simulink model "TCMSSystem"  (R2019b)
settings: configuration reference "ConfigSet_TCMSSystem_Reference" (kept outside this file)
model workspace (MAT data in the model file):
  Prm_TCMSSystem : Simulink.Parameter (value not decoded)
  SampleTime = 0.05
symbols that are objects in the model workspace (value not decoded): Prm_TCMSSystem
undefined symbols (not defined in the file): ADDIntervention, AK1Status, AK2Status, AKContactorStatus, AllDoorsClosed, AllLeftDoorsClosed, AllRightDoorsClosed, APS1Fault, APS1Isolated, APS1OutputVoltage, APS1Status, APS2Fault, APS2Isolated, APS2OutputVoltage, APS2Status, APSKAKContactor, ASCOEnd1, ASCOEnd2, ATBMode, ATCBypassMode, ATCStatusNotOK, ATOMode, ATPLowSpeedCutoutStatus, ATPMode, AuxCompressor, BatteryCurrent, BatteryIsolationContactor, BatteryTemperature, BatteryVoltage, BCG1Fault, BCG1Isolated, BCG1IsolationFailed, BCG1OutputCurrent, BCG1Status, BCG2Fault, BCG2Isolated, BCG2OutputCurrent, BCG2Status, BCGOutputVoltage, BECU1AxleLockedWheelSet1, BECU2AxleLockedWheelSet2, BECUFaulty, BECUMajorFault, BECUMinorFault, BECUStatus, BIC1Inside, BIC1Outside, BIC2Inside, BIC2Outside, Bogie, Bogie1WSPStatus, Bogie2WSPStatus, BogieFaulty, BogieIsolationStatus, BogieSupportedMass, BrakeCylinderPressureGauge, BrakeLoopCBTripped, BrakeLoopOpenTL, BrakeTrainLineStatus, BrakingDemand ... (+215)
libraries: TimersLib x257, simulink x137, LatchesLib x42, VectorOperationsLib x15, TestBenchLib x12, MathOperationsLib x2, FiltersLib x1
(part 7 of 16)

== system TCMSSystem/TCMSSystemPerVehicle/EnabledTCMSVehicle/TCMSTractionBraking/TractionBrakingControl/ForEachBogie ==
  BECUFault : Inport
  BogieBrakingEffortDemand : Inport  Port=2
  DisplayBogieControl : Inport  Port=3  Partition=on  PartitionDimension=1  PartitionWidth=1  PartitionOffset=0
  TractionBrakingBogieData : Inport  Port=4  Partition=on  PartitionDimension=1  PartitionWidth=1  PartitionOffset=0
  BogieIsolationStatus : Inport  Port=5  Partition=on  PartitionDimension=1  PartitionWidth=1  PartitionOffset=0
  UnitData : Inport  Port=6
  DynamicsIn : Inport  Port=7
  Bus Assignment : BusAssignment  AssignedSignals=EPBrakingDemand,TractionInhibit,EDBrakingInhibit,BogieSupportedMass,BogieIsolationStatus
  Bus Selector : BusSelector  OutputSignals=EstimatedSupportedMass
  Bus Selector1 : BusSelector  OutputSignals=TractionInhibit,EDBrakingInhibit
  Bus Selector2 : BusSelector  OutputSignals=EDBrakingEffortAchieved
  Constant : Constant  Value=0
  Constant7 : Constant  Value=0  OutDataTypeStr=Bus: BD_TCMSSystem_Out_Vehicle_Control_TractionBraking_Bogie
  For Each : ForEach  DisableCoverage=on
  Subsystem : Subsystem
  Sum : Sum  Inputs=+-
  Switch : Switch  Criteria=u2 > Threshold
  Terminator : Terminator
  BogieControl : Outport  ConcatenationDimension=1
  wires:
  TractionBrakingBogieData/1 -> Subsystem/3(EffortsAchivedPerVehicle), Bus Selector2/1, Bus Selector/1
  DisplayBogieControl/1 -> Bus Selector1/1
  Constant7/1 -> Bus Assignment/1  "Control"
  Bus Selector1/1 -> Bus Assignment/3  "<TractionInhibit>"
  Bus Selector1/2 -> Bus Assignment/4  "<EDBrakingInhibit>"
  Bus Selector/1 -> Bus Assignment/5  "<EstimatedSupportedMass>"
  Bus Assignment/1 -> BogieControl/1  "Control"
  BECUFault/1 -> Switch/2
  Constant/1 -> Switch/1
  Switch/1 -> Bus Assignment/2
  BogieIsolationStatus/1 -> Bus Assignment/6
  UnitData/1 -> Subsystem/1(EffortsAchievedPerUnit)
  DynamicsIn/1 -> Subsystem/2(Speed)
  BogieBrakingEffortDemand/1 -> Sum/1
  Bus Selector2/1 -> Sum/2  "<EDBrakingEffortAchieved>"
  Sum/1 -> Switch/3
  Subsystem/1(SelectEPBrakeDemand) -> Terminator/1

== system TCMSSystem/TCMSSystemPerVehicle/EnabledTCMSVehicle/TCMSTractionBraking/TractionBrakingControl/NonCabTWsAssignment ==
  TractionForce : Inport
  TractionBrakingTrainWireSource : Inport  Port=2
  EstimatedMass : Inport  Port=3
  Bus Assignment1 : BusAssignment  AssignedSignals=EstimatedMass,TractionForce
  Control : Outport
  wires:
  TractionBrakingTrainWireSource/1 -> Bus Assignment1/1
  EstimatedMass/1 -> Bus Assignment1/2
  Bus Assignment1/1 -> Control/1  "Control"
  TractionForce/1 -> Bus Assignment1/3

== system TCMSSystem/TCMSSystemPerVehicle/EnabledTCMSVehicle/TCMSTractionBraking/TractionBrakingControl/Subsystem ==
  <EstimatedSupportedMass> : Inport  Partition=on  PartitionDimension=1  PartitionWidth=1  PartitionOffset=0
  Bus Selector1 : BusSelector  OutputSignals=EstimatedSupportedMass
  For Each : ForEach  DisableCoverage=on
  EstimatedMassPerVehicle : Outport  ConcatenationDimension=1
  wires:
  <EstimatedSupportedMass>/1 -> Bus Selector1/1
  Bus Selector1/1 -> EstimatedMassPerVehicle/1  "<EstimatedSupportedMass>"

== system TCMSSystem/TCMSSystemPerVehicle/EnabledTCMSVehicle/TCMSTractionBraking/TractionBrakingControl/Subsystem1 ==
  In1 : Inport  Partition=on  PartitionDimension=1  PartitionWidth=1  PartitionOffset=0
  Bus Selector7 : BusSelector  OutputSignals=SpeedSensorFault
  For Each : ForEach  DisableCoverage=on
  <SpeedSensorFault> : Outport  ConcatenationDimension=1
  wires:
  In1/1 -> Bus Selector7/1
  Bus Selector7/1 -> <SpeedSensorFault>/1  "<SpeedSensorFault>"

== system TCMSSystem/TCMSSystemPerVehicle/EnabledTCMSVehicle/TCMSTractionBraking/TractionBrakingControl/Subsystem15 ==
  Fault : Inport
  ClearCond : Inport  Port=2
  Data Type Conversion : DataTypeConversion
  SR Latch - Reset Priority : LatchesLib/SR Latch - Reset Priority  initial_condition=0
      settings: SourceProductName=Latches
  Trig : Outport
  wires:
  Fault/1 -> SR Latch - Reset Priority/1
  SR Latch - Reset Priority/1 -> Data Type Conversion/1
  ClearCond/1 -> SR Latch - Reset Priority/2
  Data Type Conversion/1 -> Trig/1

== system TCMSSystem/TCMSSystemPerVehicle/EnabledTCMSVehicle/TCMSTractionBraking/TractionBrakingControl/Subsystem2 ==
  Fault : Inport
  ClearCond : Inport  Port=2
  Data Type Conversion : DataTypeConversion
  SR Latch - Reset Priority : LatchesLib/SR Latch - Reset Priority  initial_condition=0
      settings: SourceProductName=Latches
  Trig : Outport
  wires:
  Data Type Conversion/1 -> Trig/1
  ClearCond/1 -> SR Latch - Reset Priority/2
  SR Latch - Reset Priority/1 -> Data Type Conversion/1
  Fault/1 -> SR Latch - Reset Priority/1

== system TCMSSystem/TCMSSystemPerVehicle/EnabledTCMSVehicle/TCMSTractionBraking/TractionBrakingControl/Subsystem3 ==
  In1 : Inport  Partition=on  PartitionDimension=1  PartitionWidth=1  PartitionOffset=0
  Bus Selector7 : BusSelector  OutputSignals=TCUSlideDetected,TCUSlipDetected
  For Each : ForEach  DisableCoverage=on
  Logical Operator : Logic  Operator=OR  AllPortsSameDT=off  OutDataTypeStr=boolean
  SlipSlideDetected : Outport  ConcatenationDimension=1
  wires:
  Bus Selector7/1 -> Logical Operator/1  "<TCUSlideDetected>"
  In1/1 -> Bus Selector7/1
  Logical Operator/1 -> SlipSlideDetected/1
  Bus Selector7/2 -> Logical Operator/2  "<TCUSlipDetected>"

== system TCMSSystem/TCMSSystemPerVehicle/EnabledTCMSVehicle/TCMSTractionBraking/TractionBrakingControl/Subsystem4 ==
  In1 : Inport
  Bus Selector9 : BusSelector  OutputSignals=Bogie1IsolationCmd,Bogie2IsolationCmd
  Mux : Mux  Inputs=2
  Out1 : Outport
  wires:
  Bus Selector9/1 -> Mux/1  "<Bogie1IsolationCmd>"
  Bus Selector9/2 -> Mux/2  "<Bogie2IsolationCmd>"
  In1/1 -> Bus Selector9/1
  Mux/1 -> Out1/1

== system TCMSSystem/TCMSSystemPerVehicle/EnabledTCMSVehicle/TCMSTractionBraking/TractionBrakingDataExtract/Subsystem ==
  BogieData : Inport  Partition=on  PartitionDimension=1  PartitionWidth=1  PartitionOffset=0
  Bus Selector1 : BusSelector  OutputSignals=TCUStatus
  For Each : ForEach  DisableCoverage=on
  <TCUStatus> : Outport  ConcatenationDimension=1
  wires:
  Bus Selector1/1 -> <TCUStatus>/1  "<TCUStatus>"
  BogieData/1 -> Bus Selector1/1

== system TCMSSystem/TCMSSystemPerVehicle/EnabledTCMSVehicle/TCMSTractionBraking/TractionBrakingDataExtract/TCMSTractionBogie ==
  TractionBogieSignals : Inport  Partition=on  PartitionDimension=1  PartitionWidth=1  PartitionOffset=0
  PneumaticsBogieSignals : Inport  Port=2  Partition=on  PartitionDimension=1  PartitionWidth=1  PartitionOffset=0
  Bus Assignment : BusAssignment  AssignedSignals=TCUStatus,BogieFaulty,TractionNotIsolated,EDBrakeNotIsolated,TCUSlideDetected,TCUSlipDetected,TractiveEffortAchieved,EDBrakingEffortAchieved,TractiveEffortPossible,EDBrakingEffortPossible,TractionPower,EDBrakingPower,TractivePowerPossible,EDBrakingPowerPossible,MotorSpeeds,ASPressureSwitchStatus,EstimatedSupportedMass
  Bus Selector : BusSelector  OutputSignals=TCUStatus,BogieFaulty,TractionNotIsolated,EDBrakeNotIsolated,TCUSlideDetected,TCUSlipDetected,TractiveEffortAchieved,EDBrakingEffortAchieved,TractiveEffortPossible,EDBrakingEffortPossible,TractionPower,EDBrakingPower,TractivePowerPossible,EDBrakingPowerPossible,MotorSpeeds
  Bus Selector1 : BusSelector  OutputSignals=AirSuspensionSwitchStatus,AirSuspensionLoadPressure
  Constant : Constant  Value=Prm_TCMSSystem.LoadCompensationMasses
  Constant1 : Constant  Value=Prm_TCMSSystem.LoadCompensationPressures
  Constant7 : Constant  Value=0  OutDataTypeStr=Bus: BD_TCMSSystem_Out_Vehicle_Display_TractionBraking_Bogie
  Data Type Conversion{,1..14} (15 alike) : DataTypeConversion  OutDataTypeStr=double
  For Each : ForEach  DisableCoverage=on
  Lookup Table Dynamic : simulink/Lookup Tables/Lookup Table Dynamic  LookUpMeth=Interpolation-Use End Values  OutDataType=fixdt('double')  OutScaling=[]  OutputDataTypeScalingMode=Specify via dialog  OutDataTypeStr=double  DoSatur=off
      settings: SourceProductName=Simulink
  TCMSBogieData : Outport  ConcatenationDimension=1
  BogieTractiveEffortAchieved : Outport  Port=2  ConcatenationDimension=1
  BogieEDBrakingEffortAchieved : Outport  Port=3  ConcatenationDimension=1
  BogieTractiveEffortPossible : Outport  Port=4  ConcatenationDimension=1
  BogieEDBrakingEffortPossible : Outport  Port=5  ConcatenationDimension=1
  BogieTractivePowerAchieved : Outport  Port=6  ConcatenationDimension=1
  BogieEDBrakingPowerAchieved : Outport  Port=7  ConcatenationDimension=1
  BogieTractivePowerPossible : Outport  Port=8  ConcatenationDimension=1
  BogieEDBrakingPowerPossible : Outport  Port=9  ConcatenationDimension=1
  EstimatedBogieSupportedMass : Outport  Port=10  ConcatenationDimension=1
  TractionBogieAvailable : Outport  Port=11  ConcatenationDimension=1
  EDBrakingBogieAvailable : Outport  Port=12  ConcatenationDimension=1
  BogieFaulty : Outport  Port=13  ConcatenationDimension=1
  wires:
  Data Type Conversion3/1 -> Bus Assignment/6
  Bus Selector/15 -> Data Type Conversion8/1  "<MotorSpeeds>"
  Bus Selector/5 -> Data Type Conversion3/1  "<TCUSlideDetected>"
  Data Type Conversion10/1 -> BogieTractivePowerPossible/1, Bus Assignment/14
  Bus Selector/1 -> Data Type Conversion7/1  "<TCUStatus>"
  TractionBogieSignals/1 -> Bus Selector/1
  Bus Selector/10 -> Data Type Conversion13/1  "<EDBrakingEffortPossible>"
  Data Type Conversion13/1 -> Bus Assignment/11, BogieEDBrakingEffortPossible/1
  Bus Selector/13 -> Data Type Conversion10/1  "<TractivePowerPossible>"
  Bus Selector/12 -> Data Type Conversion11/1  "<EDBrakingPower>"
  Bus Selector/14 -> Data Type Conversion9/1  "<EDBrakingPowerPossible>"
  Bus Selector/6 -> Data Type Conversion2/1  "<TCUSlipDetected>"
  Data Type Conversion5/1 -> Bus Assignment/4, TractionBogieAvailable/1
  Bus Selector/11 -> Data Type Conversion12/1  "<TractionPower>"
  Bus Selector/4 -> Data Type Conversion4/1  "<EDBrakeNotIsolated>"
  Data Type Conversion9/1 -> BogieEDBrakingPowerPossible/1, Bus Assignment/15
  Data Type Conversion12/1 -> BogieTractivePowerAchieved/1, Bus Assignment/12
  Data Type Conversion2/1 -> Bus Assignment/7
  Bus Selector/9 -> Data Type Conversion14/1  "<TractiveEffortPossible>"
  Data Type Conversion14/1 -> Bus Assignment/10, BogieTractiveEffortPossible/1
  Data Type Conversion/1 -> Bus Assignment/9, BogieEDBrakingEffortAchieved/1
  Constant7/1 -> Bus Assignment/1  "Display"
  Bus Selector/8 -> Data Type Conversion/1  "<EDBrakingEffortAchieved>"
  Data Type Conversion8/1 -> Bus Assignment/16
  Bus Selector/3 -> Data Type Conversion5/1  "<TractionNotIsolated>"
  Bus Selector/2 -> Data Type Conversion6/1  "<BogieFaulty>"
  Data Type Conversion7/1 -> Bus Assignment/2
  Data Type Conversion6/1 -> BogieFaulty/1, Bus Assignment/3
  Bus Selector/7 -> Data Type Conversion1/1  "<TractiveEffortAchieved>"
  Bus Assignment/1 -> TCMSBogieData/1  "Display"
  Data Type Conversion1/1 -> Bus Assignment/8, BogieTractiveEffortAchieved/1
  Data Type Conversion4/1 -> EDBrakingBogieAvailable/1, Bus Assignment/5
  Data Type Conversion11/1 -> Bus Assignment/13, BogieEDBrakingPowerAchieved/1
  PneumaticsBogieSignals/1 -> Bus Selector1/1
  Bus Selector1/2 -> Lookup Table Dynamic/1  "<AirSuspensionLoadPressure>"
  Constant1/1 -> Lookup Table Dynamic/2
  Constant/1 -> Lookup Table Dynamic/3
  Lookup Table Dynamic/1 -> Bus Assignment/18, EstimatedBogieSupportedMass/1
  Bus Selector1/1 -> Bus Assignment/17  "<AirSuspensionSwitchStatus>"

== system TCMSSystem/TCMSSystemPerVehicle/EnabledTCMSVehicle/TCMSTractionBraking/TractionBrakingDisplay/BrakeScreen ==
  note: Instead of making the fault on bogie level, we only change
      | the icon at bogie level to make it simpler.
  note: Added as per BEML requirements
  note: BrakeScreen
  note: Isolation status 0 means not isolated.
  note: BECU Status is currently mapped to
      | TCUStatus(via PropulsionEnabled)
      | which is actually TCU Power
  BusIn : Inport
  In Bus Element14 : Inport  Port=2  PortName=TractionBrakingTW  Element=HoldingBrakeStatus
  In Bus Element16 : Inport  Port=2  PortName=TractionBrakingTW  Element=EstimatedMass
  In Bus Element9 : Inport  Port=3  PortName=IOControl  Element=EPIC
  In Bus Element12 : Inport  Port=3  PortName=IOControl  Element=SR
  In Bus Element13 : Inport  Port=4  PortName=TractionVehicleData  Element=EstimatedMass
  In Bus Element1 : Inport  Port=5  PortName=TractionOnBogieData
  In Bus Element17 : Inport  Port=6  PortName=BrakingSystem  Element=BrakingForce
  In Bus Element2 : Inport  Port=7  PortName=ElectricalSignals  Element=BCUPower
  In Bus Element3 : Inport  Port=8  PortName=Faults  Element=DynamicBrakeCutOut
  In Bus Element4 : Inport  Port=8  PortName=Faults  Element=BECUMajorFault
  In Bus Element5 : Inport  Port=8  PortName=Faults  Element=BECUMajorFaultWired
  In Bus Element7 : Inport  Port=9  PortName=VehicleFaults  Element=BECU1ServiceBrakeFailure
  In Bus Element8 : Inport  Port=9  PortName=VehicleFaults  Element=BECU1EmergencyBrakeFailure
  In Bus Element10 : Inport  Port=9  PortName=VehicleFaults  Element=BECU2EmergencyBrakeFailure
  In Bus Element6 : Inport  Port=9  PortName=VehicleFaults  Element=WSPActiveBogie1
  In Bus Element : Inport  Port=9  PortName=VehicleFaults  Element=BECU2MinorFault
  In Bus Element15 : Inport  Port=9  PortName=VehicleFaults  Element=BECULowRPressure
  In Bus Element18 : Inport  Port=9  PortName=VehicleFaults  Element=BECU2CarLoadPressureLow
  In Bus Element11 : Inport  Port=9  PortName=VehicleFaults  Element=BECU1CarLoadPressureLow
  AND : Logic  AllPortsSameDT=off  OutDataTypeStr=boolean
  Bus Assignment9 : BusAssignment  AssignedSignals=HoldingBrakeStatus,EPICIsolationStatus,RPRESSIsolationStatus,CarWeight,TotalWeight,Bogie1WSPStatus,Bogie2WSPStatus,EPBrakeDelivered,EDBrakeRequested,BECUStatus,BECUMinorFault,BECUMajorFault,EDCutoutStatus,DynamicBrakeCutoutDueToSlide
  Data Type Conversion{1..10} (10 alike) : DataTypeConversion
  Demux : Demux  Outputs=2
  For Each Subsystem : Subsystem  TreatAsAtomicUnit=on
  Logical Operator : Logic  Operator=OR  Inputs=4  AllPortsSameDT=off  OutDataTypeStr=boolean
  Logical Operator1 : Logic  Operator=NOT  AllPortsSameDT=off  OutDataTypeStr=boolean
  Logical Operator2 : Logic  Operator=NOT  AllPortsSameDT=off  OutDataTypeStr=boolean
  Logical Operator3 : Logic  Operator=NOT  AllPortsSameDT=off  OutDataTypeStr=boolean
  Logical Operator5 : Logic  Operator=OR  Inputs=1  AllPortsSameDT=off  OutDataTypeStr=boolean
  NOT : Logic  Operator=NOT  AllPortsSameDT=off  OutDataTypeStr=boolean
  OR : Logic  Inputs=1  AllPortsSameDT=off  OutDataTypeStr=boolean
  OR1 : Logic  Operator=OR  Inputs=5  AllPortsSameDT=off  OutDataTypeStr=boolean
  OR2 : Logic  AllPortsSameDT=off  OutDataTypeStr=boolean
  BusOut : Outport
  tag scope: SlipDetected=scoped
  wires:
  Bus Assignment9/1 -> BusOut/1
  BusIn/1 -> Bus Assignment9/1
  In Bus Element14/1 -> Data Type Conversion2/1
  Data Type Conversion2/1 -> Bus Assignment9/2
  Data Type Conversion1/1 -> Bus Assignment9/4
  In Bus Element12/1 -> Logical Operator2/1
  Logical Operator1/1 -> Data Type Conversion5/1
  Data Type Conversion5/1 -> Bus Assignment9/3
  In Bus Element9/1 -> Logical Operator1/1
  Logical Operator2/1 -> Data Type Conversion1/1
  In Bus Element13/1 -> Bus Assignment9/5
  In Bus Element16/1 -> Bus Assignment9/6
  For Each Subsystem/2(SlipDetected) -> Logical Operator5/1
  Logical Operator5/1 -> [SlipDetected]
  In Bus Element1/1 -> For Each Subsystem/1(In1)
  Demux/1 -> Bus Assignment9/7
  For Each Subsystem/1(SlideDetected) -> Data Type Conversion4/1
  Demux/2 -> OR2/1
  In Bus Element17/1 -> Bus Assignment9/9
  [EDBrakeRequested] -> Bus Assignment9/10
  Data Type Conversion10/1 -> Bus Assignment9/12
  Data Type Conversion6/1 -> Bus Assignment9/11
  In Bus Element2/1 -> Data Type Conversion6/1
  For Each Subsystem/3(EDBrakeAvailable) -> OR/1
  OR/1 -> NOT/1
  Data Type Conversion3/1 -> Bus Assignment9/14
  NOT/1 -> Data Type Conversion3/1, AND/1
  Data Type Conversion4/1 -> Demux/1
  In Bus Element3/1 -> AND/2
  AND/1 -> Data Type Conversion7/1
  Data Type Conversion7/1 -> Bus Assignment9/15
  OR1/1 -> Data Type Conversion8/1
  In Bus Element4/1 -> OR1/1
  In Bus Element5/1 -> OR1/2
  Data Type Conversion8/1 -> Bus Assignment9/13
  In Bus Element7/1 -> OR1/3
  In Bus Element8/1 -> OR1/4
  In Bus Element10/1 -> OR1/5
  In Bus Element6/1 -> Logical Operator3/1
  Logical Operator3/1 -> OR2/2
  OR2/1 -> Data Type Conversion9/1
  Data Type Conversion9/1 -> Bus Assignment9/8
  In Bus Element18/1 -> Logical Operator/3
  In Bus Element15/1 -> Logical Operator/2
  In Bus Element/1 -> Logical Operator/1
  Logical Operator/1 -> Data Type Conversion10/1
  In Bus Element11/1 -> Logical Operator/4

== system TCMSSystem/TCMSSystemPerVehicle/EnabledTCMSVehicle/TCMSTractionBraking/TractionBrakingDisplay/HVScreen ==
  note: HighVoltageScreen
  In Bus Element5 : Inport  PortName=BusIn
  In Bus Element1 : Inport  Port=2  PortName=ElectricalSignals  Element=UW_VCB
  In Bus Element : Inport  Port=2  PortName=ElectricalSignals  Element=VCBI_KAKContactorCI
  In Bus Element27 : Inport  Port=3  PortName=TractionBrakingUW  Element=CI_K_AK_Status
  Bus Assignment9 : BusAssignment  AssignedSignals=CIStatus,CIKAKContactor
  Data Type Conversion7 : DataTypeConversion
  Logical Operator : Logic  Operator=OR  AllPortsSameDT=off  OutDataTypeStr=boolean
  Display : Outport
  wires:
  In Bus Element5/1 -> Bus Assignment9/1
  Bus Assignment9/1 -> Display/1  "Display"
  In Bus Element1/1 -> Bus Assignment9/2
  Data Type Conversion7/1 -> Bus Assignment9/3
  Logical Operator/1 -> Data Type Conversion7/1
  In Bus Element27/1 -> Logical Operator/1
  In Bus Element/1 -> Logical Operator/2

== system TCMSSystem/TCMSSystemPerVehicle/EnabledTCMSVehicle/TCMSTractionBraking/TractionBrakingDisplay/OperatingandOtherScreen ==
  note: OperatingandOtherScreen
  BusIn : Inport
  In Bus Element2 : Inport  Port=2  PortName=TCMSSystemVehicleConfig
  In Bus Element : Inport  Port=3  PortName=ElectricalSignals
  In Bus Element21 : Inport  Port=4  PortName=TractionUnitData
  In Bus Element5 : Inport  Port=5  PortName=TractionVehicleData
  In Bus Element15 : Inport  Port=6  PortName=TractionBrakingTW  Element=TCMSSpeedLimit
  Abs : Abs
  Bus Assignment : BusAssignment  AssignedSignals=ForwardDirection,ReverseDirection,TrainSpeed,ZeroSpeed,TractionOn,BrakeOn,TractionSafe,UnitTractiveEffortAchieved,UnitTractiveEffortPossible,UnitEDBrakingEffortAchieved,UnitEDBrakingEffortPossible,UnitTractivePower,UnitTractivePowerPossible,UnitEDBrakingPower,UnitEDBrakingPowerPossible,VehicleTractiveEffortPossible,VehicleEDBrakingEffortAchieved,VehicleEDBrakingEffortPossible,VehicleTractivePower,VehicleTractivePowerPossible,VehicleEDBrakingPower,VehicleEDBrakingPowerPossible,VehicleTractiveEffortAchieved,TractiveEffort,TCMSSpeedLimit
  Bus Selector : BusSelector  OutputSignals=TractiveEffortPossible,EDBrakingEffortAchieved,EDBrakingEffortPossible,TractivePowerAchieved,TractivePowerPossible,EDBrakingPowerAchieved,EDBrakingPowerPossible,TractiveEffortAchieved
  Bus Selector1 : BusSelector  OutputSignals=ForwardDirection,ReverseDirection,Speedometer,ZeroSpeed,TractionOn,BrakeOn,TractionSafe,UnitTractiveEffortAchieved,UnitEDBrakingEffortAchieved,UnitTractiveEffortPossible,UnitEDBrakingEffortPossible,UnitTractivePowerAchieved,UnitEDBrakingPowerAchieved,UnitTractivePowerPossible,UnitEDBrakingPowerPossible
  CabUnitDisplay : Subsystem
  BusOut : Outport
  wires:
  Bus Selector1/6 -> Bus Assignment/7  "<BrakeOn>"
  BusIn/1 -> Bus Assignment/1  "Display"
  Bus Selector1/10 -> Bus Assignment/11  "<UnitTractiveEffortPossible>"
  Bus Selector1/3 -> Bus Assignment/4  "<Speedometer>"
  Bus Selector/6 -> Bus Assignment/22  "<EDBrakingPowerAchieved>"
  Bus Selector1/12 -> Bus Assignment/13  "<UnitTractivePowerAchieved>"
  Bus Assignment/1 -> BusOut/1
  Bus Selector/1 -> Bus Assignment/17  "<TractiveEffortPossible>"
  Bus Selector1/15 -> Bus Assignment/16  "<UnitEDBrakingPowerPossible>"
  Bus Selector1/7 -> Bus Assignment/8  "<TractionSafe>"
  Bus Selector1/2 -> Bus Assignment/3  "<ReverseDirection>"
  Bus Selector1/5 -> Bus Assignment/6  "<TractionOn>"
  Bus Selector1/14 -> Bus Assignment/15  "<UnitTractivePowerPossible>"
  Bus Selector1/8 -> Bus Assignment/9  "<UnitTractiveEffortAchieved>"
  Bus Selector1/1 -> Bus Assignment/2  "<ForwardDirection>"
  Bus Selector/4 -> Bus Assignment/20  "<TractivePowerAchieved>"
  Bus Selector1/11 -> Bus Assignment/12  "<UnitEDBrakingEffortPossible>"
  Bus Selector/2 -> Bus Assignment/18  "<EDBrakingEffortAchieved>"
  Bus Selector/3 -> Bus Assignment/19  "<EDBrakingEffortPossible>"
  CabUnitDisplay/1(CabUnitDisplay) -> Bus Selector1/1
  Bus Selector/7 -> Bus Assignment/23  "<EDBrakingPowerPossible>"
  Bus Selector1/13 -> Bus Assignment/14  "<UnitEDBrakingPowerAchieved>"
  Bus Selector1/9 -> Bus Assignment/10  "<UnitEDBrakingEffortAchieved>"
  Bus Selector1/4 -> Bus Assignment/5  "<ZeroSpeed>"
  Bus Selector/8 -> Abs/1  "<TractiveEffortAchieved>"
  Bus Selector/5 -> Bus Assignment/21  "<TractivePowerPossible>"
  In Bus Element2/1 -> CabUnitDisplay/1(TCMSConfig)
  In Bus Element/1 -> CabUnitDisplay/2(ElectricalSignals)
  In Bus Element21/1 -> CabUnitDisplay/3(TractionUnitData)
  In Bus Element5/1 -> Bus Selector/1
  Abs/1 -> Bus Assignment/25, Bus Assignment/24
  In Bus Element15/1 -> Bus Assignment/26

== system TCMSSystem/TCMSSystemPerVehicle/EnabledTCMSVehicle/TCMSTractionBraking/TractionBrakingDisplay/PropulsionScreen ==
  note: PropulsionScreen
  BusIn : Inport
  In Bus Element24 : Inport  Port=2  PortName=TractionBrakingUnitData  Element=PropulsionFault
  In Bus Element26 : Inport  Port=2  PortName=TractionBrakingUnitData  Element=PropulsionEnabled
  In Bus Element8 : Inport  Port=2  PortName=TractionBrakingUnitData  Element=PropulsionActive
  In Bus Element18 : Inport  Port=3  PortName=TractionSystem  Element=TCU_KStatus
  In Bus Element19 : Inport  Port=3  PortName=TractionSystem  Element=TCU_AKStatus
  In Bus Element20 : Inport  Port=3  PortName=TractionSystem  Element=FilterVoltage
  In Bus Element1 : Inport  Port=3  PortName=TractionSystem  Element=Bogie
  In Bus Element : Inport  Port=4  PortName=TractionOnBogieData
  In Bus Element4 : Inport  Port=5  PortName=ElectricalFB  Element=CIIsolated
  In Bus Element9 : Inport  Port=5  PortName=ElectricalFB  Element=CIIsolated
  In Bus Element5 : Inport  Port=5  PortName=ElectricalFB  Element=CabActive
  In Bus Element3 : Inport  Port=6  PortName=VehicleFault  Element=CIFailure
  In Bus Element10 : Inport  Port=6  PortName=VehicleFault  Element=LineConverterIGBTFailure
  In Bus Element2 : Inport  Port=7  PortName=CBTC  Element=RollbackDetected
  In Bus Element6 : Inport  Port=8  PortName=TractionTW  Element=HTERequired
  In Bus Element7 : Inport  Port=8  PortName=TractionTW  Element=WashModeActive
  In Bus Element11 : Inport  Port=8  PortName=TractionTW  Element=ShuntModeActive
  In Bus Element12 : Inport  Port=8  PortName=TractionTW  Element=ATPLowSpeedCutoutModeActive
  Bus Assignment9 : BusAssignment  AssignedSignals=PropulsionActive,PropulsionFault,CIFault,PropulsionIsolated,PropulsionEnableStatus,KContactorStatus,AKContactorStatus,FilterVoltage,EDBrakeStatus,HeavyWheelSlipDetected,RollbackDetected,HTERequired,WashingModeStatus,CIIsolated,ShuntModeStatus,ATPLowSpeedCutoutStatus
  Data Type Conversion{1..6} (6 alike) : DataTypeConversion
  For Each Subsystem : Subsystem  TreatAsAtomicUnit=on
  Logical Operator : Logic  Operator=OR  Inputs=3  AllPortsSameDT=off  OutDataTypeStr=boolean
  Logical Operator1 : Logic  AllPortsSameDT=off  OutDataTypeStr=boolean
  Logical Operator2 : Logic  Operator=NOT  AllPortsSameDT=off  OutDataTypeStr=boolean
  Logical Operator3 : Logic  AllPortsSameDT=off  OutDataTypeStr=boolean
  OR : Logic  Inputs=1  AllPortsSameDT=off  OutDataTypeStr=boolean
  OR1 : Logic  Operator=OR  Inputs=1  AllPortsSameDT=off  OutDataTypeStr=boolean
  BusOut : Outport
  wires:
  BusIn/1 -> Bus Assignment9/1
  Bus Assignment9/1 -> BusOut/1
  In Bus Element24/1 -> Logical Operator/1
  In Bus Element4/1 -> Logical Operator2/1, Bus Assignment9/5
  In Bus Element26/1 -> Bus Assignment9/6
  In Bus Element8/1 -> Bus Assignment9/2
  In Bus Element20/1 -> Bus Assignment9/9
  Data Type Conversion2/1 -> Bus Assignment9/7
  Data Type Conversion3/1 -> Bus Assignment9/8
  In Bus Element19/1 -> Data Type Conversion3/1
  In Bus Element18/1 -> Data Type Conversion2/1
  Data Type Conversion4/1 -> Bus Assignment9/10
  OR/1 -> Data Type Conversion4/1
  For Each Subsystem/1(EDBrakeAvailable) -> OR/1
  In Bus Element/1 -> For Each Subsystem/1(In1)
  In Bus Element1/1 -> For Each Subsystem/2(In2)
  For Each Subsystem/2(HeavyWheelSlipDetected) -> OR1/1
  OR1/1 -> Data Type Conversion1/1
  Data Type Conversion1/1 -> Bus Assignment9/11
  Logical Operator/1 -> Logical Operator1/1
  In Bus Element3/1 -> Logical Operator/2
  Data Type Conversion5/1 -> Bus Assignment9/4, Bus Assignment9/3
  Logical Operator1/1 -> Data Type Conversion5/1
  Logical Operator2/1 -> Logical Operator1/2
  In Bus Element2/1 -> Bus Assignment9/12
  In Bus Element7/1 -> Bus Assignment9/14
  Logical Operator3/1 -> Data Type Conversion6/1
  In Bus Element6/1 -> Logical Operator3/2
  In Bus Element5/1 -> Logical Operator3/1
  Data Type Conversion6/1 -> Bus Assignment9/13
  In Bus Element9/1 -> Bus Assignment9/15
  In Bus Element10/1 -> Logical Operator/3
  In Bus Element11/1 -> Bus Assignment9/16
  In Bus Element12/1 -> Bus Assignment9/17

== system TCMSSystem/TCMSSystemPerVehicle/EnabledTCMSVehicle/TCMSTractionBraking/TractionBrakingDisplay/SpeedLimitationInterlockScreen ==
  note: SpeedLimitationInterlockScreen
  In Bus Element5 : Inport  PortName=BusIn
  In Bus Element9 : Inport  PortName=BusIn  Element=EDCutoutStatus
  In Bus Element : Inport  Port=2  PortName=IOControls  Element=ASCOEnd1
  In Bus Element1 : Inport  Port=2  PortName=IOControls  Element=ASCOEnd2
  In Bus Element2 : Inport  Port=2  PortName=IOControls  Element=SafetyCutoutSS
  In Bus Element3 : Inport  Port=2  PortName=IOControls  Element=MREPICEnd1
  In Bus Element4 : Inport  Port=2  PortName=IOControls  Element=MREPICEnd2
  In Bus Element7 : Inport  Port=2  PortName=IOControls  Element=SR
  In Bus Element6 : Inport  Port=3  PortName=ElectricalSignals  Element=EBApplied
  In Bus Element8 : Inport  Port=4  PortName=PneumaticTrainSum  Element=NoOfBogieIsolated
  In Bus Element11 : Inport  Port=5  PortName=DisplayControl  Element=ATPLowModeMaxSpeed
  SlipDetected : Inport  Port=6
  AND1 : Logic  Operator=OR  AllPortsSameDT=off  OutDataTypeStr=boolean
  Bus Assignment9 : BusAssignment  AssignedSignals=SpeedLimitJogMode,SpeedLimitLowSpeedCutoutMode,SpeedLimitOverrideTractionBlock,SpeedLimitBrakeFailure,SpeedLimitASDeflated,SpeedLimitASCutout,SpeedLimitBogieIsolated,SpeedLimitNoEDAvailable,SpeedLimitRPRESSIsolated,SpeedLimitEPICCutout,SpeedLimitSCSMode,SpeedLimitExcessiveSlip
  Compare To Zero : simulink/Logic and Bit Operations/Compare To Zero  relop=>  OutDataTypeStr=boolean
  Compare To Zero1 : simulink/Logic and Bit Operations/Compare To Zero  relop=>  OutDataTypeStr=boolean
  Data Type Conversion{1..3,8..12} (8 alike) : DataTypeConversion
  FIXME1 : TestBenchLib/FIXME
      settings: SourceProductName=Sydac Utilities
  Logical Operator2 : Logic  Operator=NOT  AllPortsSameDT=off  OutDataTypeStr=boolean
  Logical Operator7 : Logic  Operator=NAND  AllPortsSameDT=off  OutDataTypeStr=boolean
  Logical Operator8 : Logic  Operator=NAND  AllPortsSameDT=off  OutDataTypeStr=boolean
  NotSupported : Constant  Value=0
  Display : Outport
  wires:
  NotSupported/1 -> Bus Assignment9/2
  FIXME1/1 -> Bus Assignment9/4, Bus Assignment9/5
  Logical Operator8/1 -> Data Type Conversion12/1
  Data Type Conversion8/1 -> Bus Assignment9/9
  Data Type Conversion11/1 -> Bus Assignment9/8
  Compare To Zero/1 -> Data Type Conversion11/1
  Data Type Conversion10/1 -> Bus Assignment9/7
  Bus Assignment9/1 -> Display/1  "Display"
  Data Type Conversion12/1 -> Bus Assignment9/11
  Logical Operator7/1 -> Data Type Conversion10/1
  AND1/1 -> Data Type Conversion8/1
  Data Type Conversion9/1 -> Bus Assignment9/13
  In Bus Element1/1 -> Logical Operator7/2
  In Bus Element5/1 -> Bus Assignment9/1
  In Bus Element3/1 -> Logical Operator8/1
  In Bus Element2/1 -> Bus Assignment9/12
  In Bus Element6/1 -> AND1/1
  In Bus Element8/1 -> Compare To Zero/1
  In Bus Element/1 -> Logical Operator7/1
  SlipDetected/1 -> Data Type Conversion9/1
  In Bus Element4/1 -> Logical Operator8/2
  In Bus Element7/1 -> Logical Operator2/1
  Logical Operator2/1 -> Data Type Conversion1/1
  Data Type Conversion1/1 -> Bus Assignment9/10
  In Bus Element9/1 -> AND1/2
  Data Type Conversion2/1 -> Bus Assignment9/6
  [ASBogie1Deflated] -> Data Type Conversion2/1
  In Bus Element11/1 -> Compare To Zero1/1
  Compare To Zero1/1 -> Data Type Conversion3/1
  Data Type Conversion3/1 -> Bus Assignment9/3

== system TCMSSystem/TCMSSystemPerVehicle/LimpHomeTCMSVehicle/TCMSTractionBraking/TractionBrakingControl/CabControlsExtract ==
  TCMSConfig : Inport
  ElectricalSignals : Inport  Port=2
  DisplayControl : Inport  Port=3
  CBTCSignals : Inport  Port=4
  InputControlStates : Inport  Port=5
  PneumaticTrainSum : Inport  Port=6
  TractionCmd : Inport  Port=7
  AND : Logic  AllPortsSameDT=off  OutDataTypeStr=boolean
  Bus Selector : BusSelector  OutputSignals=CabActive
  Bus Selector1 : BusSelector  OutputSignals=HasCab
  CabActiveTrainControl : Subsystem  TreatAsAtomicUnit=on
  CabInactiveNoTrainControl : Subsystem  TreatAsAtomicUnit=on
  Data Type Conversion : DataTypeConversion  OutDataTypeStr=uint32
  If : If
  Merge : Merge
  Speed Limit Protection : Subsystem
  TractionBrakingRefCalc : Subsystem
  TractionBrakingTrainWireSource : Outport
  wires:
  Bus Selector/1 -> AND/2  "<CabActive>"
  AND/1 -> Data Type Conversion/1
  If/2 -> CabInactiveNoTrainControl/Action
  Bus Selector1/1 -> AND/1  "<HasCab>"
  ElectricalSignals/1 -> TractionBrakingRefCalc/1(ElectricalSignals), Speed Limit Protection/1(ElectricalIn), Bus Selector/1
  TCMSConfig/1 -> Bus Selector1/1
  DisplayControl/1 -> CabActiveTrainControl/1(DisplayControl)
  If/1 -> CabActiveTrainControl/Action
  Merge/1 -> TractionBrakingTrainWireSource/1  "TractionBrakingTrainWireSource"
  Data Type Conversion/1 -> If/1
  CabInactiveNoTrainControl/1(Out1) -> Merge/2
  CabActiveTrainControl/1(Out1) -> Merge/1
  InputControlStates/1 -> Speed Limit Protection/4(IOControl)
  TractionBrakingRefCalc/1(TractionCommand) -> CabActiveTrainControl/2(TractionCommand)
  TractionBrakingRefCalc/2(BrakingCommand) -> CabActiveTrainControl/3(BrakingCommand)
  CBTCSignals/1 -> Speed Limit Protection/3(CBTCIn)
  TractionBrakingRefCalc/3(HoldingBrakesStatus) -> CabActiveTrainControl/4(HoldingBrakeStatus)
  Speed Limit Protection/1(TCMSSpeedLimit) -> CabActiveTrainControl/5(TCMSSpeedLimit)
  Speed Limit Protection/2(LimitActive) -> CabActiveTrainControl/6(LimitActive)
  TractionCmd/1 -> TractionBrakingRefCalc/2(In4)
  PneumaticTrainSum/1 -> Speed Limit Protection/2(PneumaticTrainSum)

== system TCMSSystem/TCMSSystemPerVehicle/LimpHomeTCMSVehicle/TCMSTractionBraking/TractionBrakingControl/CentralUnitControl ==
  In Bus Element3 : Inport  PortName=TractionTrainControl  Element=TractionCommand
  In Bus Element10 : Inport  PortName=TractionTrainControl  Element=BrakingCommand
  In Bus Element19 : Inport  PortName=TractionTrainControl  Element=Overspeed
  In Bus Element13 : Inport  Port=2  PortName=TractionUnitData  Element=EstimatedMass
  In Bus Element9 : Inport  Port=2  PortName=TractionUnitData  Element=TractiveEffortPossible
  In Bus Element14 : Inport  Port=2  PortName=TractionUnitData  Element=BrakingBogiesEquipped
  Constant : Constant  Value=Prm_TCMSSystem.TractionAccelerationTargets
  Constant1 : Constant  Value=Prm_TCMSSystem.BrakingDecelerationTargets
  Constant2 : Constant  Value=Prm_TCMSSystem.TractionBrakingDemands
  Constant3 : Constant  Value=Prm_TCMSSystem.TractionBrakingDemands
  Constant7 : Constant  Value=0
  Gain2 : Gain  Gain=100
  Logical Operator1 : Logic  Operator=NOT  AllPortsSameDT=off  OutDataTypeStr=boolean
  Lookup Table Dynamic1 : simulink/Lookup Tables/Lookup Table Dynamic  LookUpMeth=Interpolation-Use End Values  OutDataType=fixdt('double')  OutScaling=[]  OutputDataTypeScalingMode=Specify via dialog  OutDataTypeStr=double  DoSatur=off
      settings: SourceProductName=Simulink
  Lookup Table Dynamic2 : simulink/Lookup Tables/Lookup Table Dynamic  LookUpMeth=Interpolation-Use End Values  OutDataType=fixdt('double')  OutScaling=[]  OutputDataTypeScalingMode=Specify via dialog  OutDataTypeStr=double  DoSatur=off
      settings: SourceProductName=Simulink
  Product2 : Product
  Product3 : Product
  Product4 : Product  Inputs=**/
  Product7 : Product  Inputs=*/
  Saturation2 : Saturate  UpperLimit=1  LowerLimit=0
  safedivide2 : Saturate  UpperLimit=1e8  LowerLimit=eps
  safedivide3 : Saturate  UpperLimit=1e8  LowerLimit=eps
  TractionCommand : Outport
  EDBrakingCommand : Outport  Port=2
  BogieBrakingEffortDemand : Outport  Port=3
  wires:
  In Bus Element10/1 -> Lookup Table Dynamic2/1
  In Bus Element3/1 -> Lookup Table Dynamic1/1
  Constant2/1 -> Lookup Table Dynamic1/2
  Constant3/1 -> Lookup Table Dynamic2/2
  Lookup Table Dynamic2/1 -> Product3/2  "DecelerationDemand"
  Lookup Table Dynamic1/1 -> Product2/1  "AccelerationDemand"
  In Bus Element13/1 -> Product3/1, Product2/2  "UnitMass"
  Product2/1 -> Product4/1  "UnitEffortDemand"
  In Bus Element9/1 -> safedivide2/1
  Product3/1 -> Product7/1  "UnitEffortDemand"
  Product4/1 -> Saturation2/1
  Saturation2/1 -> Gain2/1
  Gain2/1 -> TractionCommand/1
  Constant7/1 -> EDBrakingCommand/1
  In Bus Element14/1 -> safedivide3/1
  Product7/1 -> BogieBrakingEffortDemand/1
  safedivide2/1 -> Product4/3
  safedivide3/1 -> Product7/2
  In Bus Element19/1 -> Logical Operator1/1
  Logical Operator1/1 -> Product4/2
  Constant/1 -> Lookup Table Dynamic1/3
  Constant1/1 -> Lookup Table Dynamic2/3

== system TCMSSystem/TCMSSystemPerVehicle/LimpHomeTCMSVehicle/TCMSTractionBraking/TractionBrakingControl/ForEachBogie ==
  note: Brake blending, EP compensates what ED cannot provide
  BogieBrakingEffortDemand : Inport
  TractionBrakingBogieData : Inport  Port=2  Partition=on  PartitionDimension=1  PartitionWidth=1  PartitionOffset=0
  Bus Assignment : BusAssignment  AssignedSignals=EPBrakingDemand,BogieSupportedMass
  Bus Selector : BusSelector  OutputSignals=EstimatedSupportedMass
  Constant7 : Constant  Value=0  OutDataTypeStr=Bus: BD_TCMSSystem_Out_Vehicle_Control_TractionBraking_Bogie
  For Each : ForEach  DisableCoverage=on
  BogieControl : Outport  ConcatenationDimension=1
  wires:
  TractionBrakingBogieData/1 -> Bus Selector/1
  Constant7/1 -> Bus Assignment/1  "Control"
  Bus Selector/1 -> Bus Assignment/3  "<EstimatedSupportedMass>"
  Bus Assignment/1 -> BogieControl/1  "Control"
  BogieBrakingEffortDemand/1 -> Bus Assignment/2

== system TCMSSystem/TCMSSystemPerVehicle/LimpHomeTCMSVehicle/TCMSTractionBraking/TractionBrakingDataExtract/Subsystem ==
  BogieData : Inport  Partition=on  PartitionDimension=1  PartitionWidth=1  PartitionOffset=0
  Bus Selector1 : BusSelector  OutputSignals=TCUStatus
  For Each : ForEach  DisableCoverage=on
  <TCUStatus> : Outport  ConcatenationDimension=1
  wires:
  Bus Selector1/1 -> <TCUStatus>/1  "<TCUStatus>"
  BogieData/1 -> Bus Selector1/1

== system TCMSSystem/TCMSSystemPerVehicle/LimpHomeTCMSVehicle/TCMSTractionBraking/TractionBrakingDataExtract/TCMSTractionBogie ==
  TractionBogieSignals : Inport  Partition=on  PartitionDimension=1  PartitionWidth=1  PartitionOffset=0
  AW0 : Constant  Value=42000
  Bus Assignment : BusAssignment  AssignedSignals=TCUStatus,BogieFaulty,TractionNotIsolated,EDBrakeNotIsolated,TCUSlideDetected,TCUSlipDetected,TractiveEffortAchieved,EDBrakingEffortAchieved,TractiveEffortPossible,EDBrakingEffortPossible,TractionPower,EDBrakingPower,TractivePowerPossible,EDBrakingPowerPossible,MotorSpeeds,EstimatedSupportedMass
  Bus Selector : BusSelector  OutputSignals=TCUStatus,BogieFaulty,TractionNotIsolated,EDBrakeNotIsolated,TCUSlideDetected,TCUSlipDetected,TractiveEffortAchieved,EDBrakingEffortAchieved,TractiveEffortPossible,EDBrakingEffortPossible,TractionPower,EDBrakingPower,TractivePowerPossible,EDBrakingPowerPossible,MotorSpeeds
  Constant7 : Constant  Value=0  OutDataTypeStr=Bus: BD_TCMSSystem_Out_Vehicle_Display_TractionBraking_Bogie
  Data Type Conversion{,1..14} (15 alike) : DataTypeConversion  OutDataTypeStr=double
  Divide : Product  Inputs=*/
  For Each : ForEach  DisableCoverage=on
  NoofBogies : Constant  Value=2
  TCMSBogieData : Outport  ConcatenationDimension=1
  BogieTractiveEffortAchieved : Outport  Port=2  ConcatenationDimension=1
  BogieEDBrakingEffortAchieved : Outport  Port=3  ConcatenationDimension=1
  BogieTractiveEffortPossible : Outport  Port=4  ConcatenationDimension=1
  BogieEDBrakingEffortPossible : Outport  Port=5  ConcatenationDimension=1
  BogieTractivePowerAchieved : Outport  Port=6  ConcatenationDimension=1
  BogieEDBrakingPowerAchieved : Outport  Port=7  ConcatenationDimension=1
  BogieTractivePowerPossible : Outport  Port=8  ConcatenationDimension=1
  BogieEDBrakingPowerPossible : Outport  Port=9  ConcatenationDimension=1
  EstimatedBogieSupportedMass : Outport  Port=10  ConcatenationDimension=1
  TractionBogieAvailable : Outport  Port=11  ConcatenationDimension=1
  EDBrakingBogieAvailable : Outport  Port=12  ConcatenationDimension=1
  BogieFaulty : Outport  Port=13  ConcatenationDimension=1
  wires:
  Data Type Conversion3/1 -> Bus Assignment/6
  Bus Selector/15 -> Data Type Conversion8/1  "<MotorSpeeds>"
  Bus Selector/5 -> Data Type Conversion3/1  "<TCUSlideDetected>"
  Data Type Conversion10/1 -> BogieTractivePowerPossible/1, Bus Assignment/14
  Bus Selector/1 -> Data Type Conversion7/1  "<TCUStatus>"
  TractionBogieSignals/1 -> Bus Selector/1
  Bus Selector/10 -> Data Type Conversion13/1  "<EDBrakingEffortPossible>"
  Data Type Conversion13/1 -> Bus Assignment/11, BogieEDBrakingEffortPossible/1
  Bus Selector/13 -> Data Type Conversion10/1  "<TractivePowerPossible>"
  Bus Selector/12 -> Data Type Conversion11/1  "<EDBrakingPower>"
  Bus Selector/14 -> Data Type Conversion9/1  "<EDBrakingPowerPossible>"
  Bus Selector/6 -> Data Type Conversion2/1  "<TCUSlipDetected>"
  Data Type Conversion5/1 -> Bus Assignment/4, TractionBogieAvailable/1
  Bus Selector/11 -> Data Type Conversion12/1  "<TractionPower>"
  Bus Selector/4 -> Data Type Conversion4/1  "<EDBrakeNotIsolated>"
  Data Type Conversion9/1 -> BogieEDBrakingPowerPossible/1, Bus Assignment/15
  Data Type Conversion12/1 -> BogieTractivePowerAchieved/1, Bus Assignment/12
  Data Type Conversion2/1 -> Bus Assignment/7
  Bus Selector/9 -> Data Type Conversion14/1  "<TractiveEffortPossible>"
  Data Type Conversion14/1 -> Bus Assignment/10, BogieTractiveEffortPossible/1
  Data Type Conversion/1 -> Bus Assignment/9, BogieEDBrakingEffortAchieved/1
  Constant7/1 -> Bus Assignment/1  "Display"
  Bus Selector/8 -> Data Type Conversion/1  "<EDBrakingEffortAchieved>"
  Data Type Conversion8/1 -> Bus Assignment/16
  Bus Selector/3 -> Data Type Conversion5/1  "<TractionNotIsolated>"
  Bus Selector/2 -> Data Type Conversion6/1  "<BogieFaulty>"
  Data Type Conversion7/1 -> Bus Assignment/2
  Data Type Conversion6/1 -> BogieFaulty/1, Bus Assignment/3
  Bus Selector/7 -> Data Type Conversion1/1  "<TractiveEffortAchieved>"
  Bus Assignment/1 -> TCMSBogieData/1  "Display"
  Data Type Conversion1/1 -> Bus Assignment/8, BogieTractiveEffortAchieved/1
  Data Type Conversion4/1 -> EDBrakingBogieAvailable/1, Bus Assignment/5
  Data Type Conversion11/1 -> Bus Assignment/13, BogieEDBrakingPowerAchieved/1
  Divide/1 -> EstimatedBogieSupportedMass/1, Bus Assignment/17
  AW0/1 -> Divide/1
  NoofBogies/1 -> Divide/2
